simulink model "zumoLoopback"  (R2014b)
settings: Solver=FixedStepDiscrete  StartTime=0.0  StopTime=inf  FixedStep=0.1  RelTol=1e-3
InitFcn:
  | zumo = comms.Bt('Adafruit EZ-Link 32b0', 1);
  | zumo.init();
libraries: simulink x1
settings Model: Creator=nrattner  LastModifiedBy=ksurende

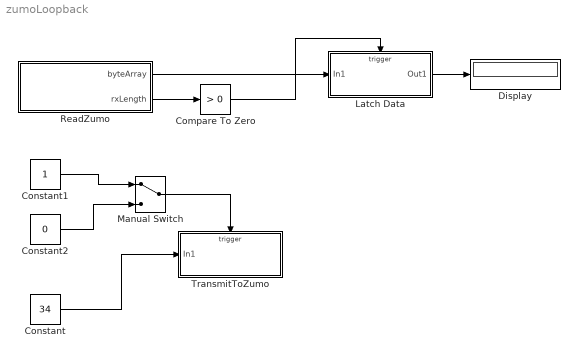
== system zumoLoopback ==
  Compare To Zero : simulink/Logic and Bit Operations/Compare To Zero  relop=>  OutDataTypeStr=boolean
  Constant : Constant  Value=34
  Constant1 : Constant  SampleTime=-1
  Constant2 : Constant  Value=0  SampleTime=-1
  Display : Display
  Latch Data : Subsystem  TreatAsAtomicUnit=on
  Manual Switch : ManualSwitch
  ReadZumo : MATLAB Function  TreatAsAtomicUnit=on
  TransmitToZumo : Subsystem  TreatAsAtomicUnit=on
  wires:
  Compare To Zero/1 -> Latch Data/Trigger
  Constant/1 -> TransmitToZumo/1(In1)
  ReadZumo/2(rxLength) -> Compare To Zero/1
  ReadZumo/1(byteArray) -> Latch Data/1(In1)
  Manual Switch/1 -> TransmitToZumo/Trigger
  Constant1/1 -> Manual Switch/1
  Constant2/1 -> Manual Switch/2
  Latch Data/1(Out1) -> Display/1

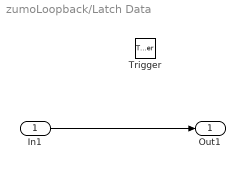
== system zumoLoopback/Latch Data ==
  In1 : Inport
  Trigger : TriggerPort
  Out1 : Outport
  wires:
  In1/1 -> Out1/1

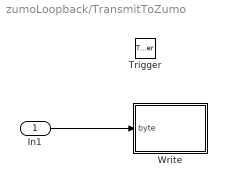
== system zumoLoopback/TransmitToZumo ==
  In1 : Inport
  Trigger : TriggerPort  TriggerType=either
  Write : MATLAB Function  TreatAsAtomicUnit=on
  wires:
  In1/1 -> Write/1(byte)

== matlab function zumoLoopback/TransmitToZumo/Write ==
  data: byte input
function write(byte)
%#codegen

coder.extrinsic('comms.writeWrapper')
comms.writeWrapper(byte,uint8(1),'Adafruit EZ-Link 32b0', 1);

== matlab function zumoLoopback/ReadZumo ==
  data: byteArray output; rxLength output
function [byteArray, rxLength] = read()
%#codegen

coder.extrinsic('comms.readWrapper');

byteArray = uint8(0);
rxLength = 0;
[byteArray,rxLength] = comms.readWrapper(1,'Adafruit EZ-Link 32b0', 1);

end
